simulink model "Pendulum_SMC"  (R2018a)
settings: Solver=VariableStepAuto  StartTime=0.0  StopTime=40  MaxStep=0.001  RelTol=1e-3
settings Model: Creator=Dell  LastModifiedBy=Dell
settings DataIOCC: ReturnWorkspaceOutputs=on
settings DebuggingCC: SFMachineParentedDataDiag=error
settings SFSimCC: SimUseLocalCustomCode=on
settings RTWCC: RTWUseLocalCustomCode=on

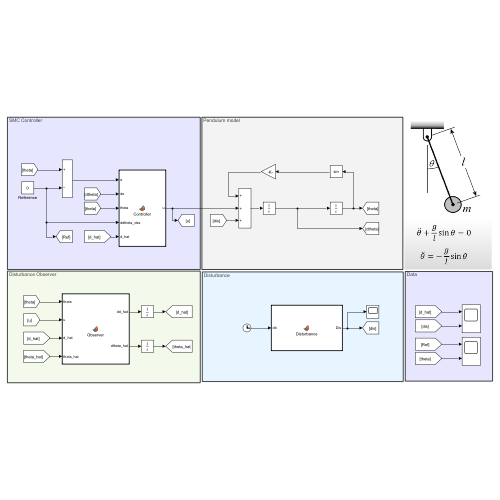
[thumbnail: Simulink's stored preview of the top-level diagram]
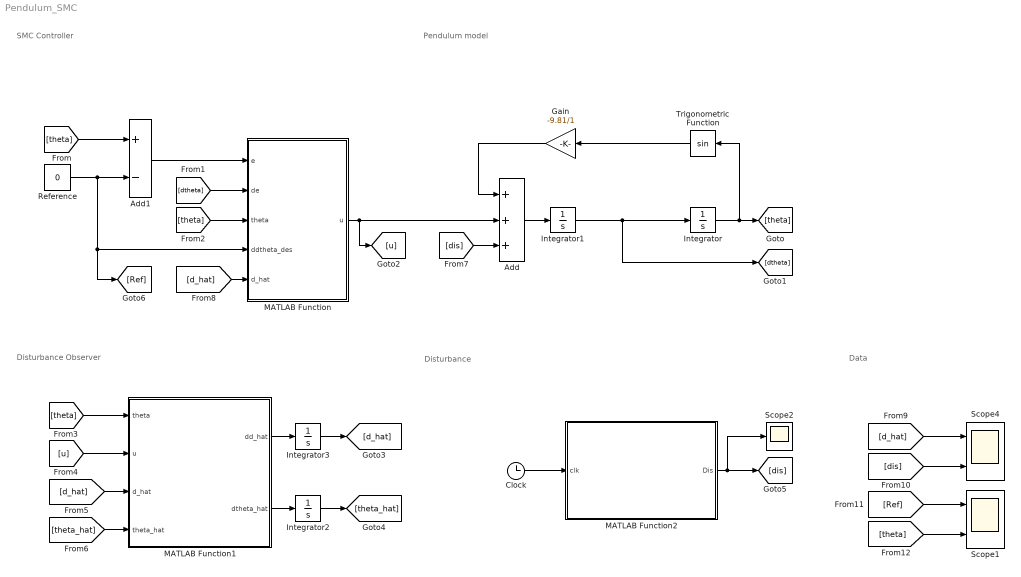
== system Pendulum_SMC ==
  note: Data
  note: Disturbance
  note: Disturbance Observer
  note: Pendulum model
  note: SMC Controller
  Add : Sum  Inputs=+++
  Add1 : Sum  Inputs=+-
  Clock : Clock
  Gain : Gain  Gain=-9.81/1
  Integrator : Integrator  InitialCondition=0.5
  Integrator1 : Integrator
  Integrator2 : Integrator  InitialCondition=0.5
  Integrator3 : Integrator
  MATLAB Function : MATLAB Function  TreatAsAtomicUnit=on
  MATLAB Function1 : MATLAB Function  TreatAsAtomicUnit=on
  MATLAB Function2 : MATLAB Function  TreatAsAtomicUnit=on
  Reference : Constant  Value=0  SampleTime=-1
  Scope1 : Scope  NumInputPorts=2
  Scope2 : Scope
  Scope4 : Scope  NumInputPorts=2
  Trigonometric Function : Trigonometry
  wires:
  Integrator/1 -> Trigonometric Function/1, [theta]
  Gain/1 -> Add/1
  Integrator1/1 -> Integrator/1, [dtheta]
  Trigonometric Function/1 -> Gain/1
  Add/1 -> Integrator1/1
  Reference/1 -> [Ref], MATLAB Function/4(ddtheta_des), Add1/2
  [theta] -> Add1/1
  Add1/1 -> MATLAB Function/1(e)
  [dtheta] -> MATLAB Function/2(de)
  [theta] -> MATLAB Function/3(theta)
  [theta] -> MATLAB Function1/1(theta)
  [u] -> MATLAB Function1/2(u)
  MATLAB Function1/2(dtheta_hat) -> Integrator2/1
  MATLAB Function1/1(dd_hat) -> Integrator3/1
  Integrator3/1 -> [d_hat]
  [d_hat] -> MATLAB Function1/3(d_hat)
  Integrator2/1 -> [theta_hat]
  [theta_hat] -> MATLAB Function1/4(theta_hat)
  Clock/1 -> MATLAB Function2/1(clk)
  [dis] -> Add/3
  MATLAB Function2/1(Dis) -> Scope2/1, [dis]
  [d_hat] -> Scope4/1
  [dis] -> Scope4/2
  [Ref] -> Scope1/1
  [theta] -> Scope1/2
  [d_hat] -> MATLAB Function/5(d_hat)
  MATLAB Function/1(u) -> Add/2, [u]

== matlab function Pendulum_SMC/MATLAB Function1 ==
  data: theta input; dd_hat output; dtheta_hat output; u input; d_hat input; theta_hat input
function [dd_hat,dtheta_hat] = Observer(theta,u,d_hat,theta_hat)
%%%%%%%%%%%%%%%%%% params %%%%%%%%%%%%%%%%%%%%%
g=9.81;    l=1;
lambda1=0.8; lambda2=0.4; sigma1=0.001;
%%%%%%%%%%%%%%%%%%%%%%%%%%%%%%%%%%%%%%%%%%%%%%%

m=-lambda1*sqrt(abs(theta_hat-theta))*sign(theta_hat-theta)+d_hat;
dtheta_hat=(-g/l)*sin(theta)+u+m;
dd_hat= -lambda2*sign(d_hat-m)-sigma1*d_hat;

== matlab function Pendulum_SMC/MATLAB Function ==
  data: e input; u output; de input; theta input; ddtheta_des input; d_hat input
function u = Controller(e,de,theta, ddtheta_des, d_hat)
%%%%%%%%%%%% Params %%%%%%%%%%%%%%%%%%%%%
lambda=1;nu=0.4;
g=9.81;l=1;
%%%%%%%%%%%%%%%%%%%%%%%%%%%%%%%%%%%%%%%%%

S=de+lambda*e;
u =(g/l)*sin(theta)+ddtheta_des-lambda*de-nu*tanh(S/0.01)-d_hat;

== matlab function Pendulum_SMC/MATLAB Function2 ==
  data: clk input; Dis output
function Dis = Disturbance(clk)

Dis = 0.2*sin(0.4*clk)+0.4*sin(clk);
